simulink model "NL_sys"  (R2019b)
settings: Solver=VariableStepAuto  StartTime=0.0  StopTime=20  RelTol=1e-3
undefined symbols (not defined in the file): g, gain, J, l, m, Mcart, n, Noise, theta
libraries: simulink x1
settings Model: Creator=huojiaxi  LastModifiedBy=huojiaxi

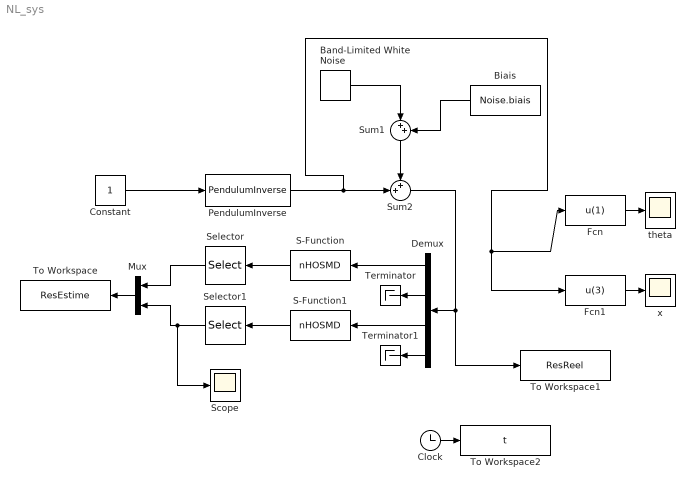
== system NL_sys ==
  Band-Limited White Noise : simulink/Sources/Band-Limited White Noise  Cov=Noise.power  Ts=Noise.sampling  seed=Noise.seed
  Biais : Constant  Value=Noise.biais
  Clock : Clock
  Constant : Constant
  Demux : Demux
  Fcn : Fcn  Expr=u(1)
  Fcn1 : Fcn  Expr=u(3)
  Mux : Mux  Inputs=2
  PendulumInverse : S-Function  FunctionName=PendulumInverse  Parameters=Mcart,m,l,g,J  SFunctionDeploymentMode=off  EnableBusSupport=off
  S-Function : S-Function  FunctionName=nHOSMD  Parameters=n,gain,theta  SFunctionDeploymentMode=off  EnableBusSupport=off
  S-Function1 : S-Function  FunctionName=nHOSMD  Parameters=n,gain,theta  SFunctionDeploymentMode=off  EnableBusSupport=off
  Scope : Scope
  Selector : Selector  InputPortWidth=n+1  IndexOptions=Index vector (dialog)  Indices=[1 2]  OutputSizes=1
  Selector1 : Selector  InputPortWidth=n+1  IndexOptions=Index vector (dialog)  Indices=[1 2]  OutputSizes=1
  Sum1 : Sum  Inputs=|++
  Sum2 : Sum  Inputs=++|
  Terminator : Terminator
  Terminator1 : Terminator
  To Workspace : ToWorkspace  VariableName=ResEstime  SampleTime=-1
  To Workspace1 : ToWorkspace  VariableName=ResReel  SampleTime=-1
  To Workspace2 : ToWorkspace  VariableName=t  SampleTime=-1
  theta : Scope
  x : Scope
  wires:
  Constant/1 -> PendulumInverse/1
  Fcn/1 -> theta/1
  Fcn1/1 -> x/1
  Demux/2 -> Terminator/1
  Demux/4 -> Terminator1/1
  Demux/1 -> S-Function/1
  Demux/3 -> S-Function1/1
  S-Function1/1 -> Selector1/1
  S-Function/1 -> Selector/1
  Mux/1 -> To Workspace/1
  Clock/1 -> To Workspace2/1
  Selector/1 -> Mux/1
  Selector1/1 -> Mux/2, Scope/1
  Sum1/1 -> Sum2/1
  Biais/1 -> Sum1/2
  Band-Limited White Noise/1 -> Sum1/1
  PendulumInverse/1 -> Fcn/1, Fcn1/1, Sum2/2
  Sum2/1 -> To Workspace1/1, Demux/1
